simulink model "control_04_rate"  (R2020a)
settings: Solver=FixedStepAuto  StartTime=0.0  StopTime=10.0  RelTol=1e-3
model workspace (MAT data in the model file):
  chi = 0.7
  omega = 100
  tau = 0.05
libraries: discretizing x9, simulink x3
settings Model: OrderedModelArguments=off  Creator=Julius  LastModifiedBy=Julius
settings OptimizationCC: DefaultUnderspecifiedDataType=single

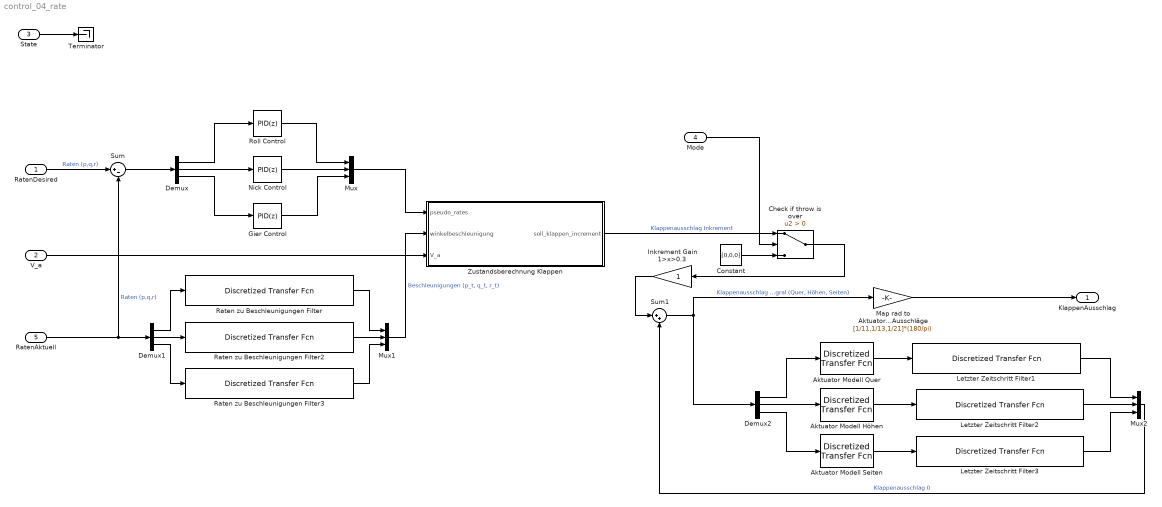
== system control_04_rate ==
  RatenDesired : Inport  OutDataTypeStr=single  PortDimensions=3
  V_a : Inport  Port=2  OutDataTypeStr=single
  State : Inport  Port=3  OutDataTypeStr=Bus: fmBus
  Mode : Inport  Port=4  OutDataTypeStr=int8
  RatenAktuell : Inport  Port=5  OutDataTypeStr=single
  Aktuator Modell Höhen : discretizing/Discretized Transfer Fcn  Numerator=[1]  Denominator=[(tau) 1]  AbsTol=auto  SampleTime=0.01  method=zoh  Wc=1
      settings: SourceProductBaseCode=SL
  Aktuator Modell Quer : discretizing/Discretized Transfer Fcn  Numerator=[1]  Denominator=[(tau) 1]  AbsTol=auto  SampleTime=0.01  method=zoh  Wc=1
      settings: SourceProductBaseCode=SL
  Aktuator Modell Seiten : discretizing/Discretized Transfer Fcn  Numerator=[1]  Denominator=[(tau) 1]  AbsTol=auto  SampleTime=0.01  method=zoh  Wc=1
      settings: SourceProductBaseCode=SL
  Check if throw is over : Switch  Criteria=u2 > Threshold
  Constant : Constant  Value=[0,0,0]  OutDataTypeStr=single
  Demux : Demux  Outputs=3
  Demux1 : Demux  Outputs=3
  Demux2 : Demux  Outputs=3
  Gier Control : simulink/Continuous/PID Controller  Controller=PID  Form=Parallel  TimeDomain=Discrete-time  UseExternalTs=off  SampleTime=0.0100000000000000002  IntegratorMethod=Forward Euler  FilterMethod=Forward Euler  ControllerParametersSource=internal  P=8  I=0.000000000000000  D=0.000000000000000  UseFilter=on  N=63.212055882855765  TunerSelectOption=Transfer Function Based (PID Tuner App)  InitialConditionSource=internal  InitialConditionForIntegrator=0  InitialConditionForFilter=0  DifferentiatorICPrevScaledInput=0  ExternalReset=none  TrackingMode=off  Kt=1  LimitOutput=off  UpperSaturationLimit=inf  LowerSaturationLimit=-inf  LinearizeAsGain=on  AntiWindupMode=none  Kb=1  POutMin=[]  POutMax=[]  IOutMin=[]  IOutMax=[]  DOutMin=[]  DOutMax=[]  NOutMin=[]  NOutMax=[]  SumOutMin=[]  SumOutMax=[]  SaturationOutMin=[]  SaturationOutMax=[]  PParamMin=[]  PParamMax=[]  IParamMin=[]  IParamMax=[]  DParamMin=[]  DParamMax=[]  NParamMin=[]  NParamMax=[]  KbParamMin=[]  KbParamMax=[]  KtParamMin=[]  KtParamMax=[]  KbOutMin=[]  KbOutMax=[]  KtOutMin=[]  KtOutMax=[]  IntegratorOutMin=[]  IntegratorOutMax=[]  FilterOutMin=[]  FilterOutMax=[]  SumI1OutMin=[]  SumI1OutMax=[]  SumI2OutMin=[]  SumI2OutMax=[]  SumI3OutMin=[]  SumI3OutMax=[]  SumI4OutMin=[]  SumI4OutMax=[]  SumDOutMin=[]  SumDOutMax=[]  DifferentiatorOutMin=[]  DifferentiatorOutMax=[]  FilterDiffOutCoefMin=[]  FilterDiffOutCoefMax=[]  ReciprocalOutMin=[]  ReciprocalOutMax=[]  SumDenOutMin=[]  SumDenOutMax=[]  SumNumOutMin=[]  SumNumOutMax=[]  DivideOutMin=[]  DivideOutMax=[]  UdiffTsProdOutMin=[]  UdiffTsProdOutMax=[]  NTsProdOutMin=[]  NTsProdOutMax=[]  UintegralTsProdOutMin=[]  UintegralTsProdOutMax=[]  UngainTsProdOutMin=[]  UngainTsProdOutMax=[]  IntegratorContinuousStateAttributes=''  IntegratorStateMustResolveToSignalObject=off  IntegratorRTWStateStorageClass=Auto  FilterContinuousStateAttributes=''  FilterStateMustResolveToSignalObject=off  FilterRTWStateStorageClass=Auto  ParallelPVariant=InternalParameters  IdealPVariant=Disabled  IVariant=InternalParameters  DVariant=InternalParameters  IntegratorVariant=Discrete  SatVariant=Disabled  AWVariant=Passthrough  PCopyVariant=Disabled  TRVariant=Disabled  FdbkBlocksVariant=Forward  IdealPFdbkVariant=Disabled  SatFdbkVariant=Disabled  DerivativeFilterVariant=ForwardEulerFilter  NVariant=InternalParameters  NCopyVariant=Disabled  FilterICVariant=InternalICsFilter  IntegratorICVariant=InternalICs  ExternalResetVariant=Disabled  TRSumVariant=Passthrough  SumFdbkVariant=Disabled  SumVariant=Sum_PID  TsampFilterVariant=InternalTs  TsampNgainVariant=Passthrough  TsampIntegralVariant=Passthrough
  Inkrement Gain 1>x>0.3 : Gain
  Letzter Zeitschritt Filter1 : discretizing/Discretized Transfer Fcn  Numerator=[(omega)^2]  Denominator=[1 2*(chi)*(omega) (omega)^2]  AbsTol=auto  SampleTime=0.01  method=zoh  Wc=1
      settings: SourceProductBaseCode=SL
  Letzter Zeitschritt Filter2 : discretizing/Discretized Transfer Fcn  Numerator=[(omega)^2]  Denominator=[1 2*(chi)*(omega) (omega)^2]  AbsTol=auto  SampleTime=0.01  method=zoh  Wc=1
      settings: SourceProductBaseCode=SL
  Letzter Zeitschritt Filter3 : discretizing/Discretized Transfer Fcn  Numerator=[(omega)^2]  Denominator=[1 2*(chi)*(omega) (omega)^2]  AbsTol=auto  SampleTime=0.01  method=zoh  Wc=1
      settings: SourceProductBaseCode=SL
  Map rad to Aktuatormodel Ausschläge : Gain  Gain=[1/11,1/13,1/21]*(180/pi)
  Mux : Mux  Inputs=3
  Mux1 : Mux  Inputs=3
  Mux2 : Mux  Inputs=3
  Nick Control : simulink/Continuous/PID Controller  Controller=PID  Form=Parallel  TimeDomain=Discrete-time  UseExternalTs=off  SampleTime=0.0100000000000000002  IntegratorMethod=Forward Euler  FilterMethod=Forward Euler  ControllerParametersSource=internal  P=8  I=0  D=0  UseFilter=on  N=63.212055882855765  TunerSelectOption=Transfer Function Based (PID Tuner App)  InitialConditionSource=internal  InitialConditionForIntegrator=0  InitialConditionForFilter=0  DifferentiatorICPrevScaledInput=0  ExternalReset=none  TrackingMode=off  Kt=1  LimitOutput=off  UpperSaturationLimit=inf  LowerSaturationLimit=-inf  LinearizeAsGain=on  AntiWindupMode=none  Kb=1  POutMin=[]  POutMax=[]  IOutMin=[]  IOutMax=[]  DOutMin=[]  DOutMax=[]  NOutMin=[]  NOutMax=[]  SumOutMin=[]  SumOutMax=[]  SaturationOutMin=[]  SaturationOutMax=[]  PParamMin=[]  PParamMax=[]  IParamMin=[]  IParamMax=[]  DParamMin=[]  DParamMax=[]  NParamMin=[]  NParamMax=[]  KbParamMin=[]  KbParamMax=[]  KtParamMin=[]  KtParamMax=[]  KbOutMin=[]  KbOutMax=[]  KtOutMin=[]  KtOutMax=[]  IntegratorOutMin=[]  IntegratorOutMax=[]  FilterOutMin=[]  FilterOutMax=[]  SumI1OutMin=[]  SumI1OutMax=[]  SumI2OutMin=[]  SumI2OutMax=[]  SumI3OutMin=[]  SumI3OutMax=[]  SumI4OutMin=[]  SumI4OutMax=[]  SumDOutMin=[]  SumDOutMax=[]  DifferentiatorOutMin=[]  DifferentiatorOutMax=[]  FilterDiffOutCoefMin=[]  FilterDiffOutCoefMax=[]  ReciprocalOutMin=[]  ReciprocalOutMax=[]  SumDenOutMin=[]  SumDenOutMax=[]  SumNumOutMin=[]  SumNumOutMax=[]  DivideOutMin=[]  DivideOutMax=[]  UdiffTsProdOutMin=[]  UdiffTsProdOutMax=[]  NTsProdOutMin=[]  NTsProdOutMax=[]  UintegralTsProdOutMin=[]  UintegralTsProdOutMax=[]  UngainTsProdOutMin=[]  UngainTsProdOutMax=[]  IntegratorContinuousStateAttributes=''  IntegratorStateMustResolveToSignalObject=off  IntegratorRTWStateStorageClass=Auto  FilterContinuousStateAttributes=''  FilterStateMustResolveToSignalObject=off  FilterRTWStateStorageClass=Auto  ParallelPVariant=InternalParameters  IdealPVariant=Disabled  IVariant=InternalParameters  DVariant=InternalParameters  IntegratorVariant=Discrete  SatVariant=Disabled  AWVariant=Passthrough  PCopyVariant=Disabled  TRVariant=Disabled  FdbkBlocksVariant=Forward  IdealPFdbkVariant=Disabled  SatFdbkVariant=Disabled  DerivativeFilterVariant=ForwardEulerFilter  NVariant=InternalParameters  NCopyVariant=Disabled  FilterICVariant=InternalICsFilter  IntegratorICVariant=InternalICs  ExternalResetVariant=Disabled  TRSumVariant=Passthrough  SumFdbkVariant=Disabled  SumVariant=Sum_PID  TsampFilterVariant=InternalTs  TsampNgainVariant=Passthrough  TsampIntegralVariant=Passthrough
  Raten zu Beschleunigungen Filter : discretizing/Discretized Transfer Fcn  Numerator=[(omega)^2 0]  Denominator=[1 2*(chi)*(omega) (omega)^2]  AbsTol=auto  SampleTime=0.01  method=zoh  Wc=0
      settings: SourceProductBaseCode=SL
  Raten zu Beschleunigungen Filter2 : discretizing/Discretized Transfer Fcn  Numerator=[(omega)^2 0]  Denominator=[1 2*(chi)*(omega) (omega)^2]  AbsTol=auto  SampleTime=0.01  method=zoh  Wc=1
      settings: SourceProductBaseCode=SL
  Raten zu Beschleunigungen Filter3 : discretizing/Discretized Transfer Fcn  Numerator=[(omega)^2 0]  Denominator=[1 2*(chi)*(omega) (omega)^2]  AbsTol=auto  SampleTime=0.01  method=zoh  Wc=1
      settings: SourceProductBaseCode=SL
  Roll Control : simulink/Continuous/PID Controller  Controller=PID  Form=Parallel  TimeDomain=Discrete-time  UseExternalTs=off  SampleTime=0.0100000000000000002  IntegratorMethod=Forward Euler  FilterMethod=Forward Euler  ControllerParametersSource=internal  P=8  I=0.000000000000000  D=0.000000000000000  UseFilter=on  N=63.212055882855765  TunerSelectOption=Transfer Function Based (PID Tuner App)  InitialConditionSource=internal  InitialConditionForIntegrator=0  InitialConditionForFilter=0  DifferentiatorICPrevScaledInput=0  ExternalReset=none  TrackingMode=off  Kt=1  LimitOutput=off  UpperSaturationLimit=inf  LowerSaturationLimit=-inf  LinearizeAsGain=on  AntiWindupMode=none  Kb=1  POutMin=[]  POutMax=[]  IOutMin=[]  IOutMax=[]  DOutMin=[]  DOutMax=[]  NOutMin=[]  NOutMax=[]  SumOutMin=[]  SumOutMax=[]  SaturationOutMin=[]  SaturationOutMax=[]  PParamMin=[]  PParamMax=[]  IParamMin=[]  IParamMax=[]  DParamMin=[]  DParamMax=[]  NParamMin=[]  NParamMax=[]  KbParamMin=[]  KbParamMax=[]  KtParamMin=[]  KtParamMax=[]  KbOutMin=[]  KbOutMax=[]  KtOutMin=[]  KtOutMax=[]  IntegratorOutMin=[]  IntegratorOutMax=[]  FilterOutMin=[]  FilterOutMax=[]  SumI1OutMin=[]  SumI1OutMax=[]  SumI2OutMin=[]  SumI2OutMax=[]  SumI3OutMin=[]  SumI3OutMax=[]  SumI4OutMin=[]  SumI4OutMax=[]  SumDOutMin=[]  SumDOutMax=[]  DifferentiatorOutMin=[]  DifferentiatorOutMax=[]  FilterDiffOutCoefMin=[]  FilterDiffOutCoefMax=[]  ReciprocalOutMin=[]  ReciprocalOutMax=[]  SumDenOutMin=[]  SumDenOutMax=[]  SumNumOutMin=[]  SumNumOutMax=[]  DivideOutMin=[]  DivideOutMax=[]  UdiffTsProdOutMin=[]  UdiffTsProdOutMax=[]  NTsProdOutMin=[]  NTsProdOutMax=[]  UintegralTsProdOutMin=[]  UintegralTsProdOutMax=[]  UngainTsProdOutMin=[]  UngainTsProdOutMax=[]  IntegratorContinuousStateAttributes=''  IntegratorStateMustResolveToSignalObject=off  IntegratorRTWStateStorageClass=Auto  FilterContinuousStateAttributes=''  FilterStateMustResolveToSignalObject=off  FilterRTWStateStorageClass=Auto  ParallelPVariant=InternalParameters  IdealPVariant=Disabled  IVariant=InternalParameters  DVariant=InternalParameters  IntegratorVariant=Discrete  SatVariant=Disabled  AWVariant=Passthrough  PCopyVariant=Disabled  TRVariant=Disabled  FdbkBlocksVariant=Forward  IdealPFdbkVariant=Disabled  SatFdbkVariant=Disabled  DerivativeFilterVariant=ForwardEulerFilter  NVariant=InternalParameters  NCopyVariant=Disabled  FilterICVariant=InternalICsFilter  IntegratorICVariant=InternalICs  ExternalResetVariant=Disabled  TRSumVariant=Passthrough  SumFdbkVariant=Disabled  SumVariant=Sum_PID  TsampFilterVariant=InternalTs  TsampNgainVariant=Passthrough  TsampIntegralVariant=Passthrough
  Sum : Sum  Inputs=|+-
  Sum1 : Sum  Inputs=|++
  Terminator : Terminator
  Zustandsberechnung Klappen : MATLAB Function  TreatAsAtomicUnit=on
  KlappenAusschlag : Outport  OutDataTypeStr=single
  wires:
  Sum/1 -> Demux/1
  Demux/3 -> Gier Control/1
  Demux/2 -> Nick Control/1
  Demux/1 -> Roll Control/1
  Gier Control/1 -> Mux/3
  Nick Control/1 -> Mux/2
  Roll Control/1 -> Mux/1
  Mux/1 -> Zustandsberechnung Klappen/1(pseudo_rates)
  Zustandsberechnung Klappen/1(soll_klappen_increment) -> Check if throw is over/1  "Klappenausschlag Inkrement"
  Sum1/1 -> Map rad to Aktuatormodel Ausschläge/1, Demux2/1  "Klappenausschlag Integral (Quer, Höhen, Seiten)"
  Aktuator Modell Quer/1 -> Letzter Zeitschritt Filter1/1
  Demux1/2 -> Raten zu Beschleunigungen Filter2/1
  Demux1/1 -> Raten zu Beschleunigungen Filter/1
  Demux1/3 -> Raten zu Beschleunigungen Filter3/1
  Raten zu Beschleunigungen Filter2/1 -> Mux1/2
  Raten zu Beschleunigungen Filter3/1 -> Mux1/3
  Raten zu Beschleunigungen Filter/1 -> Mux1/1
  Mux1/1 -> Zustandsberechnung Klappen/2(winkelbeschleunigung)  "Beschleunigungen (p_t, q_t, r_t)"
  Aktuator Modell Seiten/1 -> Letzter Zeitschritt Filter3/1
  Aktuator Modell Höhen/1 -> Letzter Zeitschritt Filter2/1
  Letzter Zeitschritt Filter2/1 -> Mux2/2
  Letzter Zeitschritt Filter3/1 -> Mux2/3
  Letzter Zeitschritt Filter1/1 -> Mux2/1
  Mux2/1 -> Sum1/2  "Klappenausschlag 0"
  Demux2/1 -> Aktuator Modell Quer/1
  Demux2/2 -> Aktuator Modell Höhen/1
  Demux2/3 -> Aktuator Modell Seiten/1
  RatenAktuell/1 -> Sum/2, Demux1/1  "Raten (p,q,r)"
  V_a/1 -> Zustandsberechnung Klappen/3(V_a)
  RatenDesired/1 -> Sum/1  "Raten (p,q,r)"
  Mode/1 -> Check if throw is over/2
  Check if throw is over/1 -> Inkrement Gain 1>x>0.3/1
  Constant/1 -> Check if throw is over/3
  State/1 -> Terminator/1
  Map rad to Aktuatormodel Ausschläge/1 -> KlappenAusschlag/1
  Inkrement Gain 1>x>0.3/1 -> Sum1/1

== matlab function control_04_rate/Zustandsberechnung Klappen ==
  data: pseudo_rates input; soll_klappen_increment output; winkelbeschleunigung input; V_a input
function soll_klappen_increment = fcn(pseudo_rates, winkelbeschleunigung, V_a)

% beschleunigung = J * derivatives * Klappenausschläge

J_vehicle = [0.2139 0 -0.0015; 0 0.2251 0; -0.0015 0 0.4362]; % Trägheitstensor
derivatives = [-0.7590, 0, 0.0081; 0, -1.0662, 0; -0.0068, 0, -0.0438]; % aerodynamic.derivatives.Cmele (Bei 0° -2° bis 2° -1.06 bis -1.07)
%derivatives = [ -0.0438, 0, 0.0081; 0, -1.0662, 0; -0.0068, 0, -0.7590]; % aerodynamic.derivatives.Cmele (Bei 0° -2° bis 2° -1.06 bis -1.07)

b_vehicle = 2.41; %(aerodynamic.b) Spannweite
S_vehicle = 0.468; %(aerodynamic.S) Flügelfläche
c_vehicle = 0.245; %(aerodynamic.chord) chord
q = 1.225/2 * V_a^2; % dyna druck

C1 = [b_vehicle, 0, 0; 0, c_vehicle, 0; 0, 0, b_vehicle];

Cm_u = q * S_vehicle * C1 * derivatives;
G = J_vehicle \ Cm_u;

soll_klappen_increment = G\(pseudo_rates - winkelbeschleunigung);
end
